simulink model "pid_simulink"  (R2021a)
settings: Solver=VariableStepAuto  StartTime=0.0  StopTime=10.0  RelTol=1e-3
undefined symbols (not defined in the file): erreur, kd, ki, kp, kt, L, R, Vfcem, Vpwm, wm
settings Model: Creator=lorm2007  LastModifiedBy=lorm2007

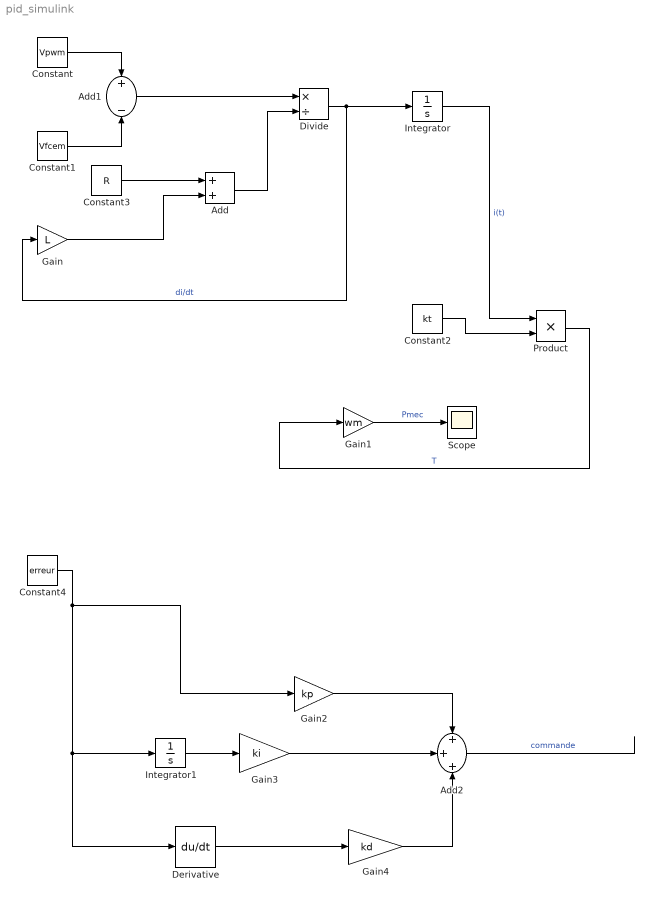
== system pid_simulink ==
  Add : Sum
  Add1 : Sum  Inputs=+-
  Add2 : Sum  Inputs=+++
  Constant : Constant  Value=Vpwm
  Constant1 : Constant  Value=Vfcem
  Constant2 : Constant  Value=kt
  Constant3 : Constant  Value=R
  Constant4 : Constant  Value=erreur
  Derivative : Derivative
  Divide : Product  Inputs=*/
  Gain : Gain  Gain=L
  Gain1 : Gain  Gain=wm
  Gain2 : Gain  Gain=kp
  Gain3 : Gain  Gain=ki
  Gain4 : Gain  Gain=kd
  Integrator : Integrator
  Integrator1 : Integrator
  Product : Product
  Scope : Scope
  wires:
  Add1/1 -> Divide/1
  Add/1 -> Divide/2
  Constant3/1 -> Add/1
  Gain/1 -> Add/2
  Product/1 -> Gain1/1  "T"
  Constant2/1 -> Product/2
  Gain1/1 -> Scope/1  "Pmec"
  Divide/1 -> Integrator/1, Gain/1  "di/dt"
  Constant1/1 -> Add1/2
  Integrator/1 -> Product/1  "i(t)"
  Constant/1 -> Add1/1
  Gain3/1 -> Add2/2
  Gain2/1 -> Add2/1
  Gain4/1 -> Add2/3
  Add2/1 -> ?  "commande"
  Derivative/1 -> Gain4/1
  Constant4/1 -> Derivative/1, Integrator1/1, Gain2/1
  Integrator1/1 -> Gain3/1
